simulink model "dft_through_inverse_GSFR"  (R2019b)
settings: Solver=VariableStepAuto  StartTime=0.0  StopTime=20  RelTol=1e-3
settings Model: Creator=ruiva  LastModifiedBy=ruiva

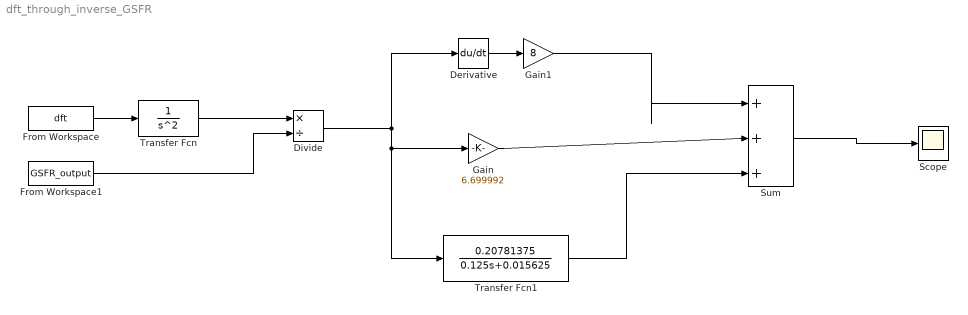
== system dft_through_inverse_GSFR ==
  Derivative : Derivative
  Divide : Product  Inputs=*/
  From Workspace : FromWorkspace  VariableName=dft  SampleTime=0
  From Workspace1 : FromWorkspace  VariableName=GSFR_output  SampleTime=0
  Gain : Gain  Gain=6.699992
  Gain1 : Gain  Gain=8
  Scope : Scope
  Sum : Sum  Inputs=|+++
  Transfer Fcn : TransferFcn  Denominator=[1 0 0]
  Transfer Fcn1 : TransferFcn  Numerator=[0.20781375]  Denominator=[0.125 0.015625]
  wires:
  From Workspace/1 -> Transfer Fcn/1
  Transfer Fcn/1 -> Divide/1
  From Workspace1/1 -> Divide/2
  Derivative/1 -> Gain1/1
  Divide/1 -> Transfer Fcn1/1, Gain/1, Derivative/1
  Sum/1 -> Scope/1
  Gain/1 -> Sum/2
  Transfer Fcn1/1 -> Sum/3
  Gain1/1 -> Sum/1
